simulink model "diagrama"  (R2020b)
settings: Solver=VariableStepAuto  StartTime=0.0  StopTime=10.0  RelTol=1e-3
settings Model: Creator=Camil  LastModifiedBy=Dalila

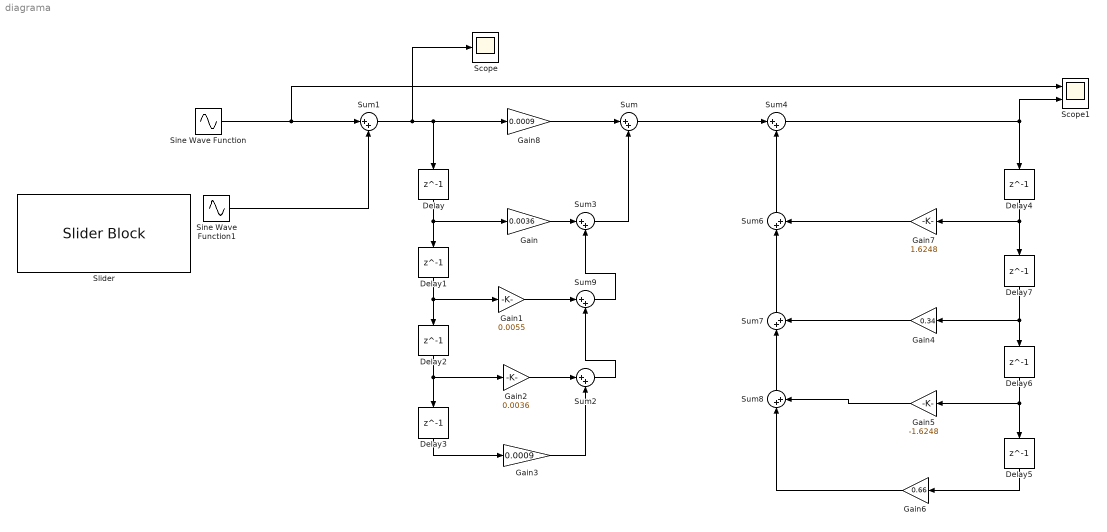
== system diagrama ==
  Delay{,1..7} (8 alike) : Delay  DelayLength=1  InitialCondition=0
  Gain : Gain  Gain=0.0036
  Gain1 : Gain  Gain=0.0055
  Gain2 : Gain  Gain=0.0036
  Gain3 : Gain  Gain=0.0009
  Gain4 : Gain  Gain=0.34
  Gain5 : Gain  Gain=-1.6248
  Gain6 : Gain  Gain=0.66
  Gain7 : Gain  Gain=1.6248
  Gain8 : Gain  Gain=0.0009
  Scope : Scope
  Scope1 : Scope  NumInputPorts=2
  Sine Wave Function : Sin  SineType=Sample based  Samples=50  SampleTime=0.001
  Sine Wave Function1 : Sin  SineType=Sample based  Amplitude=0.5  Samples=5  SampleTime=0.001
  Slider : SliderBlock  ScaleMax=5
  Sum{,1..4,6..9} (9 alike) : Sum  Inputs=|++
  wires:
  Sine Wave Function/1 -> Scope1/1, Sum1/1
  Sine Wave Function1/1 -> Sum1/2
  Sum1/1 -> Gain8/1, Delay/1, Scope/1
  Delay1/1 -> Gain1/1, Delay2/1
  Delay/1 -> Gain/1, Delay1/1
  Delay2/1 -> Gain2/1, Delay3/1
  Delay3/1 -> Gain3/1
  Gain/1 -> Sum3/1
  Gain1/1 -> Sum9/1
  Gain2/1 -> Sum2/1
  Gain3/1 -> Sum2/2
  Sum2/1 -> Sum9/2
  Sum9/1 -> Sum3/2
  Sum3/1 -> Sum/2
  Sum/1 -> Sum4/1
  Sum4/1 -> Scope1/2, Delay4/1
  Delay4/1 -> Gain7/1, Delay7/1
  Delay7/1 -> Gain4/1, Delay6/1
  Delay6/1 -> Delay5/1, Gain5/1
  Delay5/1 -> Gain6/1
  Gain7/1 -> Sum6/2
  Sum6/1 -> Sum4/2
  Sum7/1 -> Sum6/1
  Gain4/1 -> Sum7/2
  Sum8/1 -> Sum7/1
  Gain5/1 -> Sum8/2
  Gain6/1 -> Sum8/1
  Gain8/1 -> Sum/1
